simulink model "nonlinearEcuaciones"  (Simulink 7.9)
settings: Solver=ode45  StartTime=0.0  StopTime=300  MaxStep=6  RelTol=1e-3
values from neighbouring files (symbols this model uses):
  K = lqr(A,B,Q,R)    [LQR.m]    (also in bestQ.m = setK_lqr(Q_i); graficosPenduloReal.m = setK_lqr(Q_optimo))
libraries: simulink x2
settings Model: Creator=gdiazh  LastModifiedBy=root
settings OptimizationCC: InitFltsAndDblsToZero=on
settings DebuggingCC: FcnCallInpInsideContextMsg=Use local settings  StrictBusMsg=Warning
settings SFSimCC: SimParseCustomCode=off
settings GRTTargetCC: CombineOutputUpdateFcns=off  GRTInterface=on

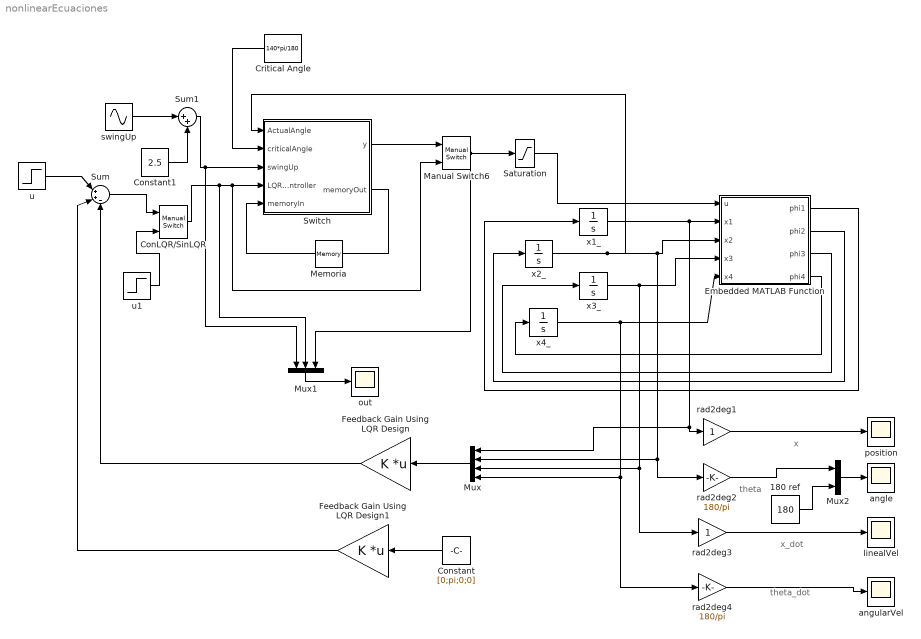
== system nonlinearEcuaciones ==
  note: x
  note: theta
  note: x_dot
  note: theta_dot
  180 ref : Constant  Value=180  VectorParams1D=off
  ConLQR/SinLQR : simulink/Signal Routing/Manual Switch  sw=1  action=0  varsize=off
  Constant : Constant  Value=[0;pi;0;0]  VectorParams1D=off
  Constant1 : Constant  Value=2.5
  Critical Angle : Constant  Value=140*pi/180
  Embedded MATLAB Function : MATLAB Function  TreatAsAtomicUnit=on
  Feedback Gain Using LQR Design : Gain  Gain=K  Multiplication=Matrix(K*u) (u vector)
  Feedback Gain Using LQR Design1 : Gain  Gain=K  Multiplication=Matrix(K*u) (u vector)
  Manual Switch6 : simulink/Signal Routing/Manual Switch  sw=0  action=0  varsize=off
  Memoria : Memory
  Mux : Mux
  Mux1 : Mux  Inputs=3
  Mux2 : Mux  Inputs=2
  Saturation : Saturate  UpperLimit=inf  LowerLimit=0
  Sum : Sum  Inputs=|++-
  Sum1 : Sum  Inputs=|++
  Switch : MATLAB Function  TreatAsAtomicUnit=on
  angle : Scope
      settings: TimeRange=0.35  YMin=180  YMax=180.007  SaveName=theta
  angularVel : Scope
      settings: YMin=-1.75e+006  YMax=1.75e+006  SaveName=angularVel
  linealVel : Scope
      settings: YMin=2e+010  YMax=5.5e+010  SaveName=linealVel
  out : Scope
      settings: TickLabels=on  YMin=0  YMax=1.4e+10  SaveName=input_u
  position : Scope
      settings: SaveName=position
  rad2deg1 : Gain  SaturateOnIntegerOverflow=on  OutDataTypeStr=Inherit: Same as input  ParamDataTypeStr=Inherit: Same as input
  rad2deg2 : Gain  Gain=180/pi  SaturateOnIntegerOverflow=on  OutDataTypeStr=Inherit: Same as input  ParamDataTypeStr=Inherit: Same as input
  rad2deg3 : Gain  SaturateOnIntegerOverflow=on  OutDataTypeStr=Inherit: Same as input  ParamDataTypeStr=Inherit: Same as input
  rad2deg4 : Gain  Gain=180/pi  SaturateOnIntegerOverflow=on  OutDataTypeStr=Inherit: Same as input  ParamDataTypeStr=Inherit: Same as input
  swingUp : Sin  Amplitude=2  Frequency=0.57*(2*pi)  SampleTime=0
  u : Step  Time=0  After=4.7/1.88  SampleTime=0
  u1 : Step  Time=0  After=4.7/1.88  SampleTime=0
  x1_ : Integrator  UpperSaturationLimit=50  LowerSaturationLimit=-50
  x2_ : Integrator  InitialCondition=190*pi/180  UpperSaturationLimit=2*pi  LowerSaturationLimit=0
  x3_ : Integrator  UpperSaturationLimit=100  LowerSaturationLimit=-100
  x4_ : Integrator  UpperSaturationLimit=100  LowerSaturationLimit=-100
  wires:
  Embedded MATLAB Function/1(phi1) -> x1_/1
  Embedded MATLAB Function/2(phi2) -> x2_/1
  Embedded MATLAB Function/3(phi3) -> x3_/1
  Embedded MATLAB Function/4(phi4) -> x4_/1
  rad2deg4/1 -> angularVel/1
  rad2deg3/1 -> linealVel/1
  rad2deg1/1 -> position/1
  x1_/1 -> Embedded MATLAB Function/2(x1), rad2deg1/1, Mux/1
  x2_/1 -> Embedded MATLAB Function/3(x2), rad2deg2/1, Mux/2, Switch/1(ActualAngle)
  x3_/1 -> Embedded MATLAB Function/4(x3), rad2deg3/1, Mux/3
  x4_/1 -> Embedded MATLAB Function/5(x4), rad2deg4/1, Mux/4
  Mux/1 -> Feedback Gain Using LQR Design/1
  Feedback Gain Using LQR Design1/1 -> Sum/2
  Constant/1 -> Feedback Gain Using LQR Design1/1
  Feedback Gain Using LQR Design/1 -> Sum/3
  Critical Angle/1 -> Switch/2(criticalAngle)
  ConLQR/SinLQR/1 -> Switch/4(LQRcontroller), Manual Switch6/2, Mux1/2
  Switch/2(memoryOut) -> Memoria/1
  Memoria/1 -> Switch/5(memoryIn)
  Manual Switch6/1 -> Mux1/3, Saturation/1
  Switch/1(y) -> Manual Switch6/1
  Sum/1 -> ConLQR/SinLQR/1
  u/1 -> Sum/1
  Mux1/1 -> out/1
  Saturation/1 -> Embedded MATLAB Function/1(u)
  Sum1/1 -> Switch/3(swingUp), Mux1/1
  Constant1/1 -> Sum1/2
  swingUp/1 -> Sum1/1
  Mux2/1 -> angle/1
  rad2deg2/1 -> Mux2/1
  180 ref/1 -> Mux2/2
  u1/1 -> ConLQR/SinLQR/2

== matlab function Switch ==
  data: y output double; ActualAngle input double; criticalAngle input double; swingUp input double; LQRcontroller input double; memoryIn input double; memoryOut output double
function [y,memoryOut] = Switch(ActualAngle, criticalAngle, swingUp, LQRcontroller,memoryIn)
%
if ((ActualAngle < criticalAngle || ActualAngle < -criticalAngle) && memoryIn ==0)
    y = swingUp;
    memoryOut = 0;
else
    memoryOut = 1;
    y = LQRcontroller;
end
end

== matlab function Embedded MATLAB Function ==
  data: u input double; x1 input double; x2 input double; x3 input double; x4 input double; phi1 output double; phi2 output double; phi3 output double; phi4 output double
function [phi1, phi2, phi3, phi4] = fcn(u, x1, x2, x3, x4)
    % This block supports the Embedded MATLAB subset.
    % See the help menu for details. 
    %Valores de los parametros
    g = 9.81;	%[m/s^2]
    M = 0.768;	%[Kg]
    m = 0.104;	%[Kg]
    l = 0.3213;	%[m]
    b = 0.05;	%[Ns/m]
    I = 0.0138;	%[Kg m^2]
    
    phi1 = x3;
    phi2 = x4;
    
    numerador = 1.88*u - 4.7 + m*l*(x4.^(2)).*sin(x2)-(b+0.548).*x3+(M+m)*g*tan(x2);
    denominador = ((M+m)*(I+m*l^2)-(m^2)*(l^2).*(cos(x2).*cos(x2)));
    
    phi3 = (I+m*l^2)*(numerador./denominador)-g*tan(x2);
    phi4 = -(numerador./denominador)*m*l.*cos(x2);
end
